simulink model "Updated"  (Simulink 6.1)
settings: Solver=ode45  StartTime=0.0  StopTime=50  RelTol=1e-3
values from neighbouring files (symbols this model uses):
  alpha = 1/2    (= 0.5)    [parameter_setup.m]
  theta1 = FrontAngle    (= 35)    [parameter_setup.m]
  theta2 = 180-FrontAngle    (= 145)    [parameter_setup.m]
  theta3 = 180+BackAngle    (= 225)    [parameter_setup.m]
  theta4 = 360-BackAngle    (= 315)    [parameter_setup.m]
  wheel_radius = 0.0254    [parameter_setup.m]
settings Model: LastModifiedBy=Binaryblade
settings DebuggingCC: SolverPrmCheckMsg=warning

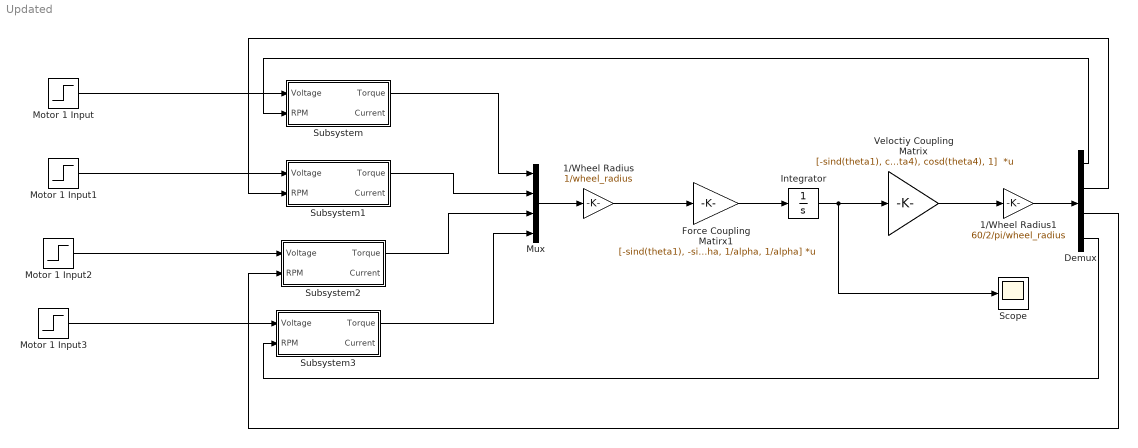
== system Updated ==
  1/Wheel Radius : Gain  Gain=1/wheel_radius
  1/Wheel Radius1 : Gain  Gain=60/2/pi/wheel_radius
  Demux : Demux
  Force Coupling Matirx1 : Gain  Gain=[-sind(theta1), -sind(theta2), -sind(theta3), -sind(theta4); cosd(theta1), cosd(theta2), cosd(theta3), cosd(theta4); 1/alpha, 1/alpha, 1/alpha, 1/alpha]  Multiplication=Matrix(K*u)
  Integrator : Integrator
  Motor 1 Input{,1..3} (4 alike) : Step  Time=5  After=12  SampleTime=0
  Mux : Mux
  Scope : Scope
  Subsystem : Subsystem
  Subsystem1 : Subsystem
  Subsystem2 : Subsystem
  Subsystem3 : Subsystem
  Veloctiy Coupling Matrix : Gain  Gain=[-sind(theta1), cosd(theta1), 1; -sind(theta2), cosd(theta2), 1; -sind(theta3), cosd(theta3), 1; -sind(theta4), cosd(theta4), 1]  Multiplication=Matrix(K*u)
  wires:
  Motor 1 Input/1 -> Subsystem/1(Voltage)
  Motor 1 Input1/1 -> Subsystem1/1(Voltage)
  Motor 1 Input2/1 -> Subsystem2/1(Voltage)
  Motor 1 Input3/1 -> Subsystem3/1(Voltage)
  Subsystem/1(Torque) -> Mux/1
  Subsystem1/1(Torque) -> Mux/2
  Subsystem2/1(Torque) -> Mux/3
  Subsystem3/1(Torque) -> Mux/4
  Mux/1 -> 1/Wheel Radius/1
  1/Wheel Radius/1 -> Force Coupling Matirx1/1
  Force Coupling Matirx1/1 -> Integrator/1
  Integrator/1 -> Veloctiy Coupling Matrix/1, Scope/1
  Veloctiy Coupling Matrix/1 -> 1/Wheel Radius1/1
  1/Wheel Radius1/1 -> Demux/1
  Demux/1 -> Subsystem/2(RPM)
  Demux/2 -> Subsystem1/2(RPM)
  Demux/3 -> Subsystem2/2(RPM)
  Demux/4 -> Subsystem3/2(RPM)

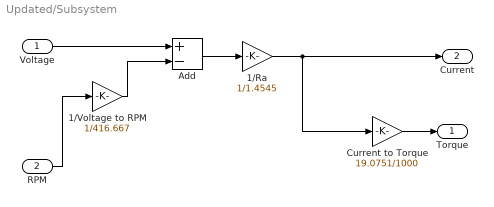
== system Updated/Subsystem ==
  Voltage : Inport  Port=1  LatchInput=off
  RPM : Inport  Port=2  LatchInput=off
  1/Ra : Gain  Gain=1/1.4545
  1/Voltage to RPM : Gain  Gain=1/416.667
  Add : Sum  Inputs=+-  OutScaling=2^-10
  Current to Torque : Gain  Gain=19.0751/1000
  Torque : Outport
  Current : Outport  Port=2
  wires:
  Voltage/1 -> Add/1
  1/Voltage to RPM/1 -> Add/2
  RPM/1 -> 1/Voltage to RPM/1
  Add/1 -> 1/Ra/1
  1/Ra/1 -> Current/1, Current to Torque/1
  Current to Torque/1 -> Torque/1

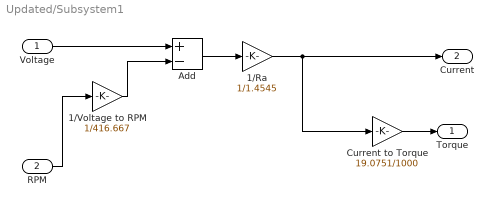
== system Updated/Subsystem1 ==
  Voltage : Inport  Port=1  LatchInput=off
  RPM : Inport  Port=2  LatchInput=off
  1/Ra : Gain  Gain=1/1.4545
  1/Voltage to RPM : Gain  Gain=1/416.667
  Add : Sum  Inputs=+-  OutScaling=2^-10
  Current to Torque : Gain  Gain=19.0751/1000
  Torque : Outport
  Current : Outport  Port=2
  wires:
  Voltage/1 -> Add/1
  1/Voltage to RPM/1 -> Add/2
  RPM/1 -> 1/Voltage to RPM/1
  Add/1 -> 1/Ra/1
  1/Ra/1 -> Current/1, Current to Torque/1
  Current to Torque/1 -> Torque/1

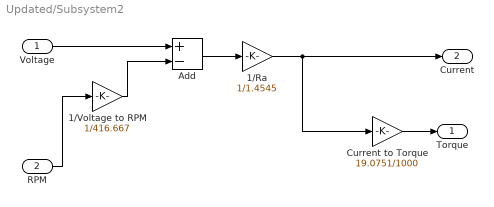
== system Updated/Subsystem2 ==
  Voltage : Inport  Port=1  LatchInput=off
  RPM : Inport  Port=2  LatchInput=off
  1/Ra : Gain  Gain=1/1.4545
  1/Voltage to RPM : Gain  Gain=1/416.667
  Add : Sum  Inputs=+-  OutScaling=2^-10
  Current to Torque : Gain  Gain=19.0751/1000
  Torque : Outport
  Current : Outport  Port=2
  wires:
  Voltage/1 -> Add/1
  1/Voltage to RPM/1 -> Add/2
  RPM/1 -> 1/Voltage to RPM/1
  Add/1 -> 1/Ra/1
  1/Ra/1 -> Current/1, Current to Torque/1
  Current to Torque/1 -> Torque/1

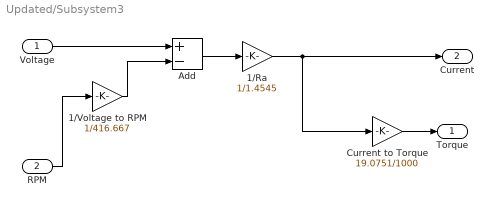
== system Updated/Subsystem3 ==
  Voltage : Inport  Port=1  LatchInput=off
  RPM : Inport  Port=2  LatchInput=off
  1/Ra : Gain  Gain=1/1.4545
  1/Voltage to RPM : Gain  Gain=1/416.667
  Add : Sum  Inputs=+-  OutScaling=2^-10
  Current to Torque : Gain  Gain=19.0751/1000
  Torque : Outport
  Current : Outport  Port=2
  wires:
  Voltage/1 -> Add/1
  1/Voltage to RPM/1 -> Add/2
  RPM/1 -> 1/Voltage to RPM/1
  Add/1 -> 1/Ra/1
  1/Ra/1 -> Current/1, Current to Torque/1
  Current to Torque/1 -> Torque/1
